simulink model "ML_UAV_3D_2"  (R2018a)
settings: Solver=ode4  StartTime=0.0  StopTime=130  FixedStep=Ts  MaxStep=2*T  MinStep=T  RelTol=1e-4
values from neighbouring files (symbols this model uses):
  Ac = 0.0331    [init_ML_UAV_3D_2.m]
  Am1_LPF = sysd.denominator{1}    [init_ML_UAV_3D_2.m]
  Am2_LPF = sysd.denominator{1}    [init_ML_UAV_3D_2.m]
  Am_coup_LPF = sysd.denominator{1}    [init_ML_UAV_3D_2.m]
  Amp_sf = 3    [init_ML_UAV_3D_2.m]
  Amp_sf_rp = 0.05*uav.m*g    [init_ML_UAV_3D_2.m]
  Bm1_LPF = sysd.numerator{1}    [init_ML_UAV_3D_2.m]
  Bm2_LPF = sysd.numerator{1}    [init_ML_UAV_3D_2.m]
  Bm_coup_LPF = sysd.numerator{1}    [init_ML_UAV_3D_2.m]
  C_S = [5;5;9]*10^-3    [init_ML_UAV_3D_2.m]
  Cd_u = 0.2    [init_ML_UAV_3D_2.m]
  dc_M_p = 6.7    [init_ML_UAV_3D_2.m]
  eps_V = 0.5    [init_ML_UAV_3D_2.m]
  g = 9.81    [init_ML_UAV_3D_2.m]
  gamma_d_p = (2*0.3/0.03*2*0.2*12/4)/10    (= 2.4)    [init_ML_UAV_3D_2.m]
  k3 = 24    [init_ML_UAV_3D_2.m]
  k4 = 0.8    [init_ML_UAV_3D_2.m]
  min_sf = 5    [init_ML_UAV_3D_2.m]
  min_sf_rp = 0.35*uav.m*g    [init_ML_UAV_3D_2.m]
  OMEGA_FILTER_OUTER = 40    [estimation.m]
  T_init = 10    [init_ML_UAV_3D_2.m]
  Tc = 1/500    (= 0.002)    [estimation.m]
  Tg = 1/ 20    (= 0.05)    [estimation.m]
  Tn = 1/500    (= 0.002)    [estimation.m]
  Ts = 1/500    (= 0.002)    [estimation.m]    (also in init_ML_UAV_3D_2.m)
  Tsc = 1/100    (= 0.01)    [estimation.m]
  Tz = 1/500    (= 0.002)    [estimation.m]
  X_GPS_offset = [0.01 0.005]    [estimation.m]
undefined symbols (not defined in the file or in its folder): Am_HPF, Am_LPF, Am_LPF2, an1, an1_v, an2, an3, Bm_HPF, Bm_LPF, Bm_LPF2, bn1, bn1_v, bn2, bn3, buoy, cable, controller, current, D_b, DiscIntNeverNeededParam, F, filters, J_u, K, kd_t, kp_t, L, Light, magnitude, MIL, Phi0, Psi0, R_b, T, Theta0, theta_q_ini, tolerences, torque_corr, uav, Vol_b, water, wave, X0_u
libraries: simulink x48, simulink_extras x10, UAV_Control x4, dspmtrx3 x2, aerolibwind2 x2
(part 6 of 6)

== system ML_UAV_3D_2/Quadrotor+buoy/6-DOF equations of motion Earth frame/azimuthal dynamics/Coupled System's azimuthal dynamics/elevation and azimuth angles dynamics in the coupled system ==
  alpha_phi_ddot : Inport
  alpha phi init : Inport  Port=2
  alpha_phi_dot init : Inport  Port=3
  reset : Inport  Port=4
  Enable : EnablePort
  " alpha" : Scope
  " alpha dot" : Scope
  " alpha dot init" : Scope
  " alpha init" : Scope
  "alpha, phi" : DiscreteIntegrator  IntegratorMethod=Integration: Backward Euler  ExternalReset=level  InitialConditionSource=external  InitialCondition=a_p_0  SampleTime=-1  ICPrevOutput=DiscIntNeverNeededParam  ICPrevScaledInput=DiscIntNeverNeededParam
  "dot(alpha, phi)" : DiscreteIntegrator  IntegratorMethod=Integration: Backward Euler  ExternalReset=level  InitialConditionSource=external  SampleTime=-1  ICPrevOutput=DiscIntNeverNeededParam  ICPrevScaledInput=DiscIntNeverNeededParam
  "reset " : Scope
  "alpha, phi " : Outport
  "alpha_dot, phi_dot" : Outport  Port=2
  wires:
  "dot(alpha, phi)"/1 -> "alpha, phi"/1, " alpha dot"/1, "alpha_dot, phi_dot"/1
  alpha_phi_ddot/1 -> "dot(alpha, phi)"/1
  "alpha, phi"/1 -> "alpha, phi "/1, " alpha"/1
  alpha_phi_dot init/1 -> " alpha dot init"/1, "dot(alpha, phi)"/3
  alpha phi init/1 -> " alpha init"/1, "alpha, phi"/3
  reset/1 -> "reset "/1, "alpha, phi"/2, "dot(alpha, phi)"/2

== system ML_UAV_3D_2/Quadrotor+buoy/6-DOF equations of motion Earth frame/azimuthal dynamics/Coupled System's azimuthal dynamics/get initial elevation and azimuth angle for the coupled dynamics ==
  "alpha, phi decoupled" : Inport
  "alpha_dot, phi_dot decoupled" : Inport  Port=2
  Trigger : TriggerPort  VariantControl=Variant
  "alpha, phi init" : Outport
  "alpha_dot, phi_dot init" : Outport  Port=2
  wires:
  "alpha, phi decoupled"/1 -> "alpha, phi init"/1
  "alpha_dot, phi_dot decoupled"/1 -> "alpha_dot, phi_dot init"/1

== system ML_UAV_3D_2/Quadrotor+buoy/6-DOF equations of motion Earth frame/azimuthal dynamics/Decoupled System's elevation and azimuth dynamics/elevation and azimuth angles to Direction Cosine Matrix Spherical to Cartesian ==
  "alpha, phi" : Inport
  -s_alpha*c_phi : Fcn  Expr=-u(1)*u(4)
  -s_alpha*s_phi : Fcn  Expr=-u(1)*u(2)
  -s_phi : Fcn  Expr=-u(2)
  Ground : Ground
  Mux : Mux  Inputs=2
  Subsystem : Subsystem
  c_alpha : Fcn  Expr=u(3)
  c_alpha*c_phi : Fcn  Expr=u(3)*u(4)
  c_alpha*s_phi : Fcn  Expr=u(3)*u(2)
  c_phi : Fcn  Expr=u(4)
  s_alpha : Fcn  Expr=u(1)
  sincos : Trigonometry  Operator=sincos
  DCM : Outport  PortDimensions=[3,3]
  wires:
  -s_alpha*c_phi/1 -> Subsystem/2(In2)
  -s_phi/1 -> Subsystem/3(In3)
  Subsystem/1(Out1) -> DCM/1
  c_alpha/1 -> Subsystem/8(In8)
  sincos/2 -> Mux/2
  s_alpha/1 -> Subsystem/7(In7)
  c_alpha*s_phi/1 -> Subsystem/4(In4)
  Ground/1 -> Subsystem/9(In9)
  Mux/1 -> c_alpha*s_phi/1, s_alpha/1, c_alpha/1, c_phi/1, -s_alpha*s_phi/1, -s_phi/1, -s_alpha*c_phi/1, c_alpha*c_phi/1
  -s_alpha*s_phi/1 -> Subsystem/5(In5)
  c_alpha*c_phi/1 -> Subsystem/1(In1)
  c_phi/1 -> Subsystem/6(In6)
  sincos/1 -> Mux/1
  "alpha, phi"/1 -> sincos/1

== system ML_UAV_3D_2/Quadrotor+buoy/6-DOF equations of motion Earth frame/azimuthal dynamics/Decoupled System's elevation and azimuth dynamics/magnitude ==
  dX : Inport
  Math Function2 : Math  Operator=square  SaturateOnIntegerOverflow=on
  Sqrt : Sqrt  SaturateOnIntegerOverflow=on
  Sum of Elements : Sum  Inputs=+
  r : Outport
  wires:
  Math Function2/1 -> Sum of Elements/1
  Sum of Elements/1 -> Sqrt/1
  dX/1 -> Math Function2/1
  Sqrt/1 -> r/1

== system ML_UAV_3D_2/Quadrotor+buoy/6-DOF equations of motion Earth frame/azimuthal dynamics/Decoupled System's elevation and azimuth dynamics/magnitude1 ==
  dX : Inport
  Math Function2 : Math  Operator=square  SaturateOnIntegerOverflow=on
  Sqrt : Sqrt  SaturateOnIntegerOverflow=on
  Sum of Elements : Sum  Inputs=+
  r : Outport
  wires:
  Sqrt/1 -> r/1
  dX/1 -> Math Function2/1
  Sum of Elements/1 -> Sqrt/1
  Math Function2/1 -> Sum of Elements/1

== system ML_UAV_3D_2/Sensors and Filters/Sensors/ Sonar (10Hz) (true elevation instead real sonar signal)/Sampler/Triggered Subsystem ==
  In1 : Inport
  Trigger : TriggerPort  VariantControl=(inherit)
  Out1 : Outport
  wires:
  In1/1 -> Out1/1

== system ML_UAV_3D_2/UAV controller/u_r_p_Lyapunov radial position2/output conditioning/Subsystem1/ur smooth lower bound, coupled ==
  u : Inport
  Manual Switch : ManualSwitch
  Mux3 : Mux  Inputs=2
  Saturation1 : Saturate  UpperLimit=inf  LowerLimit=min_sf
  apply for lower bound only : Switch  Criteria=u2 > Threshold  Threshold=Amp_sf+min_sf
  sat : Scope
  saturation function : Fcn  Expr=Amp_sf*tanh((u(1)-(Amp_sf+min_sf))/(Amp_sf)) + (Amp_sf+min_sf)
  sat(u) : Outport
  wires:
  Manual Switch/1 -> sat(u)/1
  Saturation1/1 -> Manual Switch/2
  u/1 -> saturation function/1, apply for lower bound only/2, Mux3/1, apply for lower bound only/1, Saturation1/1
  saturation function/1 -> apply for lower bound only/3, Mux3/2
  Mux3/1 -> sat/1
  apply for lower bound only/1 -> Manual Switch/1

== system ML_UAV_3D_2/UAV controller/u_r_p_Lyapunov radial position2/output conditioning/Subsystem1/ur smooth lower bound, decoupled ==
  u : Inport
  Manual Switch : ManualSwitch
  Mux3 : Mux  Inputs=2
  Saturation1 : Saturate  UpperLimit=inf  LowerLimit=min_sf_rp
  apply for lower bound only : Switch  Criteria=u2 > Threshold  Threshold=Amp_sf_rp+min_sf_rp
  sat : Scope
  saturation function : Fcn  Expr=Amp_sf_rp*tanh((u(1)-(Amp_sf_rp+min_sf_rp))/(Amp_sf_rp)) + (Amp_sf_rp+min_sf_rp)
  sat(u) : Outport
  wires:
  Manual Switch/1 -> sat(u)/1
  Saturation1/1 -> Manual Switch/2
  u/1 -> saturation function/1, apply for lower bound only/2, Mux3/1, apply for lower bound only/1, Saturation1/1
  saturation function/1 -> apply for lower bound only/3, Mux3/2
  Mux3/1 -> sat/1
  apply for lower bound only/1 -> Manual Switch/1

== system ML_UAV_3D_2/UAV controller/u_r_p_Lyapunov radial position2/output conditioning/smooth switching with memory/Enabled Subsystem1 ==
  In1 : Inport
  Enable : EnablePort
  Out1 : Outport
  wires:
  In1/1 -> Out1/1

== system ML_UAV_3D_2/UAV controller/u_r_p_Lyapunov radial position2/output conditioning/smooth switching with memory/Enabled Subsystem2 ==
  In1 : Inport
  Enable : EnablePort
  Out1 : Outport
  wires:
  In1/1 -> Out1/1

== system ML_UAV_3D_2/UAV controller/u_r_p_Lyapunov radial position2/output conditioning/smooth switching with memory/smooth switch ==
  note: if switch == 0
      | y = u2
      | elseif switch == 1
      | y = u1
      | end
  u 1 : Inport
  u 2 : Inport  Port=2
  switch : Inport  Port=3
  Constant : Constant
  Data Type Conversion : DataTypeConversion
  Low Pass Filter2 : DiscreteTransferFcn  Numerator=filters.Bm_coup_LPF  Denominator=filters.Am_coup_LPF
  Product : Product
  Product1 : Product
  Step1 : Step  SampleTime=0
  Subtract : Sum  Inputs=+-
  Sum : Sum  Inputs=|++
  "switch " : Scope
  y : Outport
  wires:
  Product/1 -> Sum/2
  Product1/1 -> Sum/1
  Low Pass Filter2/1 -> "switch "/1, Product/1, Subtract/2
  Data Type Conversion/1 -> Low Pass Filter2/1
  u 2/1 -> Product1/1
  u 1/1 -> Product/2
  switch/1 -> Data Type Conversion/1
  Sum/1 -> y/1
  Constant/1 -> Subtract/1
  Subtract/1 -> Product1/2

== system ML_UAV_3D_2/UAV controller/u_r_p_Lyapunov radial position3/output conditioning/Subsystem1/ur smooth lower bound, coupled ==
  u : Inport
  Manual Switch : ManualSwitch
  Mux3 : Mux  Inputs=2
  Saturation1 : Saturate  UpperLimit=inf  LowerLimit=min_sf
  apply for lower bound only : Switch  Criteria=u2 > Threshold  Threshold=Amp_sf+min_sf
  sat : Scope
  saturation function : Fcn  Expr=Amp_sf*tanh((u(1)-(Amp_sf+min_sf))/(Amp_sf)) + (Amp_sf+min_sf)
  sat(u) : Outport
  wires:
  Manual Switch/1 -> sat(u)/1
  Saturation1/1 -> Manual Switch/2
  u/1 -> saturation function/1, apply for lower bound only/2, Mux3/1, apply for lower bound only/1, Saturation1/1
  saturation function/1 -> apply for lower bound only/3, Mux3/2
  Mux3/1 -> sat/1
  apply for lower bound only/1 -> Manual Switch/1

== system ML_UAV_3D_2/UAV controller/u_r_p_Lyapunov radial position3/output conditioning/Subsystem1/ur smooth lower bound, decoupled ==
  u : Inport
  Manual Switch : ManualSwitch
  Mux3 : Mux  Inputs=2
  Saturation1 : Saturate  UpperLimit=inf  LowerLimit=min_sf_rp
  apply for lower bound only : Switch  Criteria=u2 > Threshold  Threshold=Amp_sf_rp+min_sf_rp
  sat : Scope
  saturation function : Fcn  Expr=Amp_sf_rp*tanh((u(1)-(Amp_sf_rp+min_sf_rp))/(Amp_sf_rp)) + (Amp_sf_rp+min_sf_rp)
  sat(u) : Outport
  wires:
  Manual Switch/1 -> sat(u)/1
  Saturation1/1 -> Manual Switch/2
  u/1 -> saturation function/1, apply for lower bound only/2, Mux3/1, apply for lower bound only/1, Saturation1/1
  saturation function/1 -> apply for lower bound only/3, Mux3/2
  Mux3/1 -> sat/1
  apply for lower bound only/1 -> Manual Switch/1

== system ML_UAV_3D_2/UAV controller/u_r_p_Lyapunov radial position3/output conditioning/smooth switching with memory/Enabled Subsystem1 ==
  In1 : Inport
  Enable : EnablePort
  Out1 : Outport
  wires:
  In1/1 -> Out1/1

== system ML_UAV_3D_2/UAV controller/u_r_p_Lyapunov radial position3/output conditioning/smooth switching with memory/Enabled Subsystem2 ==
  In1 : Inport
  Enable : EnablePort
  Out1 : Outport
  wires:
  In1/1 -> Out1/1

== system ML_UAV_3D_2/UAV controller/u_r_p_Lyapunov radial position3/output conditioning/smooth switching with memory/smooth switch ==
  note: if switch == 0
      | y = u2
      | elseif switch == 1
      | y = u1
      | end
  u 1 : Inport
  u 2 : Inport  Port=2
  switch : Inport  Port=3
  Constant : Constant
  Data Type Conversion : DataTypeConversion
  Low Pass Filter2 : DiscreteTransferFcn  Numerator=Bm_coup_LPF  Denominator=Am_coup_LPF
  Product : Product
  Product1 : Product
  Step1 : Step  SampleTime=0
  Subtract : Sum  Inputs=+-
  Sum : Sum  Inputs=|++
  "switch " : Scope
  y : Outport
  wires:
  Product/1 -> Sum/2
  Product1/1 -> Sum/1
  Low Pass Filter2/1 -> "switch "/1, Product/1, Subtract/2
  Data Type Conversion/1 -> Low Pass Filter2/1
  u 2/1 -> Product1/1
  u 1/1 -> Product/2
  switch/1 -> Data Type Conversion/1
  Sum/1 -> y/1
  Constant/1 -> Subtract/1
  Subtract/1 -> Product1/2

== system ML_UAV_3D_2/Quadrotor+buoy/6-DOF equations of motion Earth frame/azimuthal dynamics/Decoupled System's elevation and azimuth dynamics/elevation and azimuth angles to Direction Cosine Matrix Spherical to Cartesian/Subsystem ==
  In1 : Inport
  In2 : Inport  Port=2
  In3 : Inport  Port=3
  In4 : Inport  Port=4
  In5 : Inport  Port=5
  In6 : Inport  Port=6
  In7 : Inport  Port=7
  In8 : Inport  Port=8
  In9 : Inport  Port=9
  Matrix Concatenate : Concatenate  NumInputs=3  Mode=Multidimensional array  ConcatenateDimension=2
  Mux : Mux  Inputs=3
  Mux1 : Mux  Inputs=3
  Mux2 : Mux  Inputs=3
  Reshape : Reshape  OutputDimensionality=Column vector (2-D)
  Reshape1 : Reshape  OutputDimensionality=Column vector (2-D)
  Reshape2 : Reshape  OutputDimensionality=Column vector (2-D)
  Out1 : Outport
  wires:
  Reshape1/1 -> Matrix Concatenate/2
  Mux1/1 -> Reshape1/1
  Reshape/1 -> Matrix Concatenate/1
  Reshape2/1 -> Matrix Concatenate/3
  Matrix Concatenate/1 -> Out1/1
  Mux2/1 -> Reshape2/1
  In1/1 -> Mux/1
  Mux/1 -> Reshape/1
  In4/1 -> Mux/2
  In7/1 -> Mux/3
  In2/1 -> Mux1/1
  In8/1 -> Mux1/3
  In5/1 -> Mux1/2
  In3/1 -> Mux2/1
  In6/1 -> Mux2/2
  In9/1 -> Mux2/3

== matlab function ML_UAV_3D_2/Sea2/Water current ==
  data: Uc input; Us input; uc output; beta input; psi_b input; vc output; psi_w input
function [uc,vc] = fcn(Uc,Us,beta,psi_b,psi_w)

%% body frame:
% uc = Uc*cos(beta - psi_b) + sum( Us.*cos(psi_w - psi_b) );
% vc = Uc*sin(beta - psi_b) + sum( Us.*sin(psi_w - psi_b) );

%% inertial frame:
uc = Uc*cos(beta) + sum( Us.*cos(psi_w) );
vc = Uc*sin(beta) + sum( Us.*sin(psi_w) );

== matlab function ML_UAV_3D_2/Quadrotor+buoy/6-DOF equations of motion Earth frame/Coupling state/MATLAB Function ==
  data: pos_T input; is_coupled output; re_couple input; coupled input; c output
function [is_coupled,c] = fcn(pos_T, re_couple, coupled)

% persistent coupled
% if isempty(coupled) 
%     coupled = 1;
% end

if and(pos_T == 1 , coupled == 1)
    coupled = 1;
    c = 1; 
    
elseif and(pos_T == 0 , coupled == 1)
    coupled = 0;
    c = 2;
elseif and(coupled == 0 , re_couple == 0)
    coupled = 0;
    c = 3;
elseif and(coupled == 0 , re_couple == 1)
    coupled = 1;
    c = 4;
elseif and(pos_T == 0 , coupled == 0)
    coupled = 0;
    c = 5;
else
    coupled = 1;
    c = 6;
end
    
is_coupled = coupled;

== matlab function ML_UAV_3D_2/Sensors and Filters/Data processing/Estimate Attitude/Kalman Filter - Pitch ==
  settings: updateMethod=DISCRETE  sampleTime=T
  data: angle output; acc_angle input; gyro_rate input; opti_angle input; dt input
function angle   = fcn(acc_angle,gyro_rate,opti_angle,dt)
%#eml
    % a bias in the accelerometer will result in a bias in the filter
    % estimate
    Q_angle = 0.001;
    Q_gyro   = 0.001; %0.01;  %0.003
    R_angle  =  0.01;  %0.03

    
    persistent P_00;
    persistent P_01;
    persistent P_10;
    persistent P_11;
    persistent x_angle;
    persistent x_bias;
        
    if isempty(P_00)
        P_00 = 1.5*10^-4;
    end
    
    if isempty(P_01)
        P_01 = -1.4*10^-4;
    end
    if isempty(P_10)
        P_10 = -1.4*10^-4;
    end
    if isempty(P_11)
        P_11 = 11.4*10^-4;
    end
     if isempty(x_bias)
        x_bias = 0;
     end
     if isempty(x_angle)
        x_angle = 0;
     end
    
    
    % Calculate the new output
    x_angle = x_angle + dt * (gyro_rate - x_bias);%
    P_00 = P_00 -  dt * (P_10 + P_01) + Q_angle * dt;
    P_01 = P_01  - dt * P_11;
    P_10 = P_10  - dt * P_11;
    P_11 = P_11  + Q_gyro * dt;

    % Assuming H = [0.98 (effect of gyro) 0.02 (effect of acc)]
    %e = (0.97*x_angle + 0.03*acc_angle) - x_angle;
    e = (0.9*x_angle + 0.001*acc_angle + 0.099*opti_angle) - x_angle;
    S = P_00 + R_angle;
    K_0 = P_00 / S;
    K_1 = P_10 / S;

    % Correction
    x_angle = x_angle+  K_0 * e;
    x_bias  = x_bias+  K_1 * e;
    P_00 = P_00 - K_0 * P_00;
    P_01 = P_01 - K_0 * P_01;
    P_10 = P_10 - K_1 * P_00;
    P_11 = P_11 - K_1 * P_01;

    angle = x_angle;
%     P = [P_00 P_01; P_10 P_11];

== matlab function ML_UAV_3D_2/Sensors and Filters/Coupling detection by r/Coupling state/MATLAB Function ==
  data: pos_T input; is_coupled output; re_couple input; coupled input; c output
function [is_coupled,c] = fcn(pos_T, re_couple, coupled)

% persistent coupled
% if isempty(coupled) 
%     coupled = 1;
% end

if and(pos_T == 1 , coupled == 1)
    coupled = 1;
    c = 1; 
    
elseif and(pos_T == 0 , coupled == 1)
    coupled = 0;
    c = 2;
elseif and(coupled == 0 , re_couple == 0)
    coupled = 0;
    c = 3;
elseif and(coupled == 0 , re_couple == 1)
    coupled = 1;
    c = 4;
elseif and(pos_T == 0 , coupled == 0)
    coupled = 0;
    c = 5;
else
    coupled = 1;
    c = 6;
end
    
is_coupled = coupled;

== matlab function ML_UAV_3D_2/Sensors and Filters/Data processing/Estimate Position/Extrapolation - x ==
  settings: updateMethod=DISCRETE
  data: xin input; xout output; xdotin input; dt input; new input; isTracking input; x0 input
function xout = fcn(xin, xdotin, dt, new, isTracking,x0)
%#codegen

%
% Pass through input if "new" data available and OptiTrack is tracking.
% Otherwise, use linear interpolation to estimate the signal value and
% ignore the input data.
%
persistent x;

if( isempty(x) )
    x = x0;
end;

if( new == 1 && isTracking == 1 )
    x = xin;
else
    x = x+dt*xdotin;
end;

xout = x;

== matlab function ML_UAV_3D_2/Preprocessing Unit/setpoint velocity controller  ==
  settings: updateMethod=DISCRETE
  data: V_ref input; phi_bar input; Vb input; r_ref input; alpha_ref output; zb input; phi_bar_dec output; zu_ref input; D_b11 input; T_bar output
function [alpha_ref,phi_bar_dec,T_bar] = ...
    fcn(V_ref, phi_bar,Vb,r_ref,zb,zu_ref,D_b11)

% if t < 1
%     r_ref = 3; %r_0 = 3;
% else
%     r_ref = 6.7; %r_bar = 6.7;
% end

alpha_ref = asin( (zu_ref - zb)/r_ref );

xb_dot_ref = V_ref*cos(phi_bar);
yb_dot_ref = V_ref*sin(phi_bar);

% phi_bar_dec = atan2( V_ref*sin(psi_V_ref)-Vb(2), V_ref*cos(psi_V_ref)-Vb(1));
phi_bar_dec = phi_bar;

% mag2_Vb = sqrt(Vb(1)^2 + Vb(2)^2);
T_bar = D_b11*sqrt( (xb_dot_ref-Vb(1))^2 + (yb_dot_ref-Vb(2))^2 )/cos(alpha_ref);

== matlab function ML_UAV_3D_2/Sensors and Filters/Data processing/Estimate Position/Extrapolation - z ==
  settings: updateMethod=DISCRETE  sampleTime=T
  data: xin input; xout output; xdotin input; dt input; new input; isTracking input; x0 input
function xout = fcn(xin, xdotin, dt, new, isTracking,x0)
%#codegen

%
% Pass through input if "new" data available and OptiTrack is tracking.
% Otherwise, use linear interpolation to estimate the signal value and
% ignore the input data.
%
persistent x;

if( isempty(x) )
    x = x0;
end

if( new == 1 && isTracking == 1 )
    x = xin;
else
    x = x+dt*xdotin;
end

xout = x;

== matlab function ML_UAV_3D_2/UAV controller/cond1/MATLAB Function ==
  settings: updateMethod=DISCRETE
  data: r input; r_dot input; y output; coupled input; Lc input; dt input; t output
function [y,t]  = fcn(r,r_dot,coupled,Lc,dt)

persistent key
persistent timer

if isempty(key)
    key = 0;
end

if isempty(timer)
    timer = 0;
end

if (r > Lc - 0.1) && (r_dot > 0.25) && (key == 0)
    key = 1;
end

if (r < Lc - 0.12) && (r_dot < -0.1) && (key == 1)
    key = 0;
end

if (key == 1) && (coupled == 1)
    timer = timer + dt;
end

if (timer >= 1) % reset
    key = 0;
    timer = 0;
end

y = key;
t = timer;

== matlab function ML_UAV_3D_2/Preprocessing Unit/Damping Coefficient Calculation ==
  settings: updateMethod=DISCRETE
  data: Re output; V_bar input; delta_h input; h_b input; l_b input; C_S_bar output; rho input; nu input; b_11 input; D11_0 output
function [Re,C_S_bar,D11_0]  = fcn(V_bar,delta_h,h_b,l_b,rho,nu,b_11)

Re = max(abs(V_bar)*l_b/nu,0.5*10^5);

C_S_bar = 0.075/(log10(Re) -2 )^2;

D11_0 = V_bar*( max(min(delta_h+h_b/2,h_b),0)*(2*l_b) + (l_b*h_b) )...
        *0.5*rho*C_S_bar + b_11;

== matlab function ML_UAV_3D_2/UAV controller/State Machine new ==
  settings: updateMethod=DISCRETE  sampleTime=T
  data: eps input; r input; r_thr input; active output; mag_Vb2 input; psi_Vb input; V_bar0 input; c output; V_bar input; reset input
function [active,c] = fcn(eps,r, r_thr,mag_Vb2,psi_Vb, V_bar0, V_bar,reset)

persistent state
persistent is_active

if isempty(is_active) 
    state = 0;
    is_active = 0;
end

eps = abs(eps); % make sure that eps is positive.
eps_p1 = 2*eps;
eps_p2 = 2.5*eps;
eps_n1 = 1.5*eps;
eps_n2 = 2*eps;

dx_thr = 0.13;  
% deactivate the velocity controller while reset is on:
if (reset == 1)
    is_active = 0;
    % idel state
    state = 0; 
% buoy velocity is low, activate to accelerate:
elseif and( is_active == 0, mag_Vb2 <= V_bar0-eps_n1 )  
    is_active = 1;
    % accelerate flag state
    state = 1;     
 
% deactivate since velocity has gone too high or the system has
% unintentionnally decouple to prevent damage (removed for testing):
elseif and( is_active == 1 , (mag_Vb2 >= V_bar+eps_p1) ) % (r < r_thr)
    is_active = 0;
    % acceleration stop state
    state = 2;
    
% deactivate since velocity has gone too high or the system has
% unintentionnally decouple to prevent damage:
% elseif and( is_active == 1, or( (mag_Vb2 >= V_bar+eps_n1), (r < r_thr) )) % (r < r_thr)
%     is_active = 0;
%     % acceleration stop state
%     state = 3; 
end    
 
%%
c           = state;
active      =  is_active;

== matlab function ML_UAV_3D_2/Refenrence Commands/setpoint velocity controller1 ==
  settings: updateMethod=DISCRETE
  data: eps input; r input; er_thr input; V_bar_out output; phi_bar_out output; Lc0 input; c output; V0_bar input; phi0_bar input; V input
function [V_bar_out,phi_bar_out,c] = fcn(eps,r, er_thr, Lc0,...
            V0_bar,phi0_bar, V) 

persistent V0_old
if isempty(V0_old) 
    V0_old = 0;
end

eps = abs(eps); % make sure that eps is positive.

% Velocity error is low, no output.
if (V0_bar - V <  eps) && (V0_bar - V >=  0)
    V_bar_out = V0_old;
    % return previous V0
    c = 0; 
% Velocity error is high, output the velocity only if the UAV is ready.
elseif (V0_bar - V >=  eps) && (Lc0 - r < er_thr)
    V_bar_out = V0_bar;
    % follow new V0
    c = 1;     
% Velocity error is low, no output.
elseif (V0_bar - V >  -eps) && (V0_bar - V <  0)
    V_bar_out = V0_old;
    % return previous V0
    c = 2; 
% Velocity error is high, output the velocity only if the UAV is ready.
elseif (V0_bar - V <=  -eps) && (Lc0 - r < er_thr)
    V_bar_out = V0_bar;
    % follow new V0
    c = 3;
else  % Velocity error is high, but UAV is not ready
    V_bar_out = V0_old;
    c = 4;
end

% when the new reference velocity is sent to the ouptut,
% set the old reference velocity to the current reference velocty
% to be the zero point when the reference velocty changes again.
if  V_bar_out == V0_bar
    V0_old = V0_bar;
end

phi_bar_out = phi0_bar;

== matlab function ML_UAV_3D_2/UAV controller/Attitutde Control/PID control law with saturation and ff acceleration1 ==
  settings: updateMethod=DISCRETE
  data: ex input; ex_int output; u output; ex_dot input; xd_ddot input; kp input; kd input; ki input; exi_max input; u_min input; u_max input; m input; dt input; u_sat output
function [ex_int,u,u_sat] = fcn(ex,ex_dot,xd_ddot,kp,kd,ki,exi_max,u_min,u_max,m,dt)

persistent int_ex;

if isempty(int_ex)
    int_ex = 0;
end

int_ex = max(min(int_ex + ex*dt,exi_max),-exi_max);

u = m*(-kp*ex - ki*int_ex - kd*ex_dot + xd_ddot);

u_sat = max(min(u,u_max),u_min);

ex_int = int_ex;

== matlab function ML_UAV_3D_2/UAV controller/Attitutde Control/PID control law with saturation and ff acceleration ==
  settings: updateMethod=DISCRETE
  data: ex input; ex_int output; u output; ex_dot input; xd_ddot input; kp input; kd input; ki input; exi_max input; u_min input; u_max input; m input; dt input; u_sat output
function [ex_int,u,u_sat] = fcn(ex,ex_dot,xd_ddot,kp,kd,ki,exi_max,u_min,u_max,m,dt)

persistent int_ex;

if isempty(int_ex)
    int_ex = 0;
end

int_ex = max(min(int_ex + ex*dt,exi_max),-exi_max);

u = m*(-kp*ex - ki*int_ex - kd*ex_dot + xd_ddot);

u_sat = max(min(u,u_max),u_min);

ex_int = int_ex;

== matlab function ML_UAV_3D_2/UAV controller/Decoupling control signals /control signals decoupling ==
  data: ur input; u_C output; u1 output; phi_u output; theta_u output; ua input; uf input; alpha input; phi input; psi_u input; uz_min input; u1_max input; tilt_max input
function [u_C,u1,phi_u,theta_u] = fcn(ur,ua,uf,alpha,phi,psi_u,...
            uz_min,u1_max,tilt_max)

% u_C = [ux;uy;uz]
% tested for correctness

u_C = [cos(alpha)*cos(phi),  -sin(alpha)*cos(phi), -sin(phi)
       cos(alpha)*sin(phi),  -sin(alpha)*sin(phi),  cos(phi)
       sin(alpha)         ,   cos(alpha)         ,     0    ]...
      ...
      *[ur;ua;uf];

u_C(3,1) = max(uz_min,u_C(3,1)); 

     u1 = min(sqrt(u_C(1,1)^2 + u_C(2,1)^2 + u_C(3,1)^2), u1_max);
     
  phi_u = atan( (u_C(1,1)*sin(psi_u) - u_C(2,1)*cos(psi_u)) / u_C(3,1) );
  
theta_u = asin( (u_C(1,1)*cos(psi_u) + u_C(2,1)*sin(psi_u)) /u1 );

  phi_u  = tilt_max*tanh(   phi_u/tilt_max );
theta_u  = tilt_max*tanh( theta_u/tilt_max );

== matlab function ML_UAV_3D_2/UAV controller/Attitutde Control/PID control law with saturation and ff acceleration2 ==
  settings: updateMethod=DISCRETE  sampleTime=Ts
  data: ex input; ex_int output; u output; ex_dot input; xd_ddot input; kp input; kd input; ki input; exi_max input; u_min input; u_max input; m input; dt input; u_sat output
function [ex_int,u,u_sat] = fcn(ex,ex_dot,xd_ddot,kp,kd,ki,exi_max,u_min,u_max,m,dt)

persistent int_ex;

if isempty(int_ex)
    int_ex = 0;
end

int_ex = max(min(int_ex + ex*dt,exi_max),-exi_max);

u = m*(-kp*ex - ki*int_ex - kd*ex_dot + xd_ddot);

u_sat = max(min(u,u_max),u_min);

ex_int = int_ex;

== matlab function ML_UAV_3D_2/Sensors and Filters/Data processing/Estimate Attitude/Calculate Roll and Pitch (From Acceleration Data)/calc_roll_pitch ==
  data: roll_acc output; pitch_acc output; acc_body input
function [roll_acc, pitch_acc]   = fcn(acc_body)
%#eml
n = norm(acc_body,2);
if n>eps
    acc_body = -acc_body/n; 
else
    acc_body = [0 0 1]';
end

roll_acc = atan2(acc_body(2),acc_body(3));
pitch_acc = atan2( -acc_body(1), acc_body(2)*sin(roll_acc)+acc_body(3)*cos(roll_acc));

== matlab function ML_UAV_3D_2/Sensors and Filters/Data processing/Estimate Position/Kalman Filter - Height ==
  settings: updateMethod=DISCRETE  sampleTime=T
  data: height output; optitrack input; sonar_d input; dt input; x0 input
function height   = fcn(optitrack,sonar_d,dt,x0)
%#eml

     Q_sonar  = 0.1; %0.01; %0.001
     Q_optitrack   = 0.01; %0.01;  %0.003
     R_height =  0.03;  %0.03

    
    persistent P_00;
    persistent P_01;
    persistent P_10;
    persistent P_11;
    persistent x_height;
    persistent x_bias;
        
    if isempty(P_00)
        P_00 = 0;
    end
    
    if isempty(P_01)
        P_01 = 0;
    end
    if isempty(P_10)
        P_10 = 0;
    end
    if isempty(P_11)
        P_11 = 0;
    end
    if isempty(x_bias)
       x_bias = 0;
    end
    if isempty(x_height)
       x_height = x0;
    end
    
    
    % Compensate for sonar rate calculation (sonar sample rate is 10Hz)
    sonar_d_corrected = sonar_d*dt*10;  % m/s
    
    % Reject large height rate changes from sonar
    % As those are likely a result of obstacle underneath or noise
    if(abs(sonar_d_corrected) > 1 )    % max height rate (m/s)
        sonar_d_corrected = 0;
    end
    
    % Calculate the new output
    %x_height = x_height + dt * (sonar_d - x_bias); % old 
    x_height = x_height + dt * (sonar_d_corrected - x_bias);
    P_00 = P_00 -  dt * (P_10 + P_01) + Q_sonar * dt;
    P_01 = P_01  - dt * P_11;
    P_10 = P_10  - dt * P_11;
    P_11 = P_11  + Q_optitrack * dt;

    % Assuming H = [0.95 (effect of optitrack) 0.05 (effect of sonar)]
    e = (0.05*x_height + 0.95*optitrack) - x_height;
    S = P_00 + R_height;
    K_0 = P_00 / S;
    K_1 = P_10 / S;

    % Correction
    x_height = x_height+  K_0 * e;
    x_bias  = x_bias+  K_1 * e;
    P_00 = P_00 - K_0 * P_00;
    P_01 = P_01 - K_0 * P_01;
    P_10 = P_10 - K_1 * P_00;
    P_11 = P_11 - K_1 * P_01;

    height = x_height;

== matlab function ML_UAV_3D_2/Sea2/Waves (elevation and speed) ==
  data: x input; zeta_xy output; y input; z input; t input; A input; psi input; omega input; k input; epsilon input; uw output; vw output; ww output; phi_water output; theta_water output
function [zeta_xy,uw,vw,ww,phi_water,theta_water] = ...
            fcn(x,y,z,t,A,psi,omega,k,epsilon)

f = - k*x.*cos(psi) - k.*y.*sin(psi) + omega*t + epsilon;
zeta_xy = sum( A.*sin(f) );

e = exp(k*z);

uw = sum( omega.*A.*e.*sin(f).*cos(psi) );
vw = sum( omega.*A.*e.*sin(f).*sin(psi) );
ww = sum( omega.*A.*e.*cos(f) );

  phi_water = atan( sum(-A.*k.*sin(psi).*cos(f)) );

theta_water = atan( sum(-A.*k.*cos(psi).*cos(f)) );

== matlab function ML_UAV_3D_2/Refenrence Commands/referense signals selector ==
  settings: updateMethod=DISCRETE
  data: V_ref input; phi_ref input; tv_ref input; V_ref_out output; r_ref input; phi_ref_out output; zu_ref input; tr_ref input; t input; r_ref_out output; zu_ref_out output
function [V_ref_out,phi_ref_out,r_ref_out,zu_ref_out] = ...
    fcn(V_ref,phi_ref,tv_ref,r_ref,zu_ref,tr_ref,t)

persistent i j

if isempty(i)
i = 1;
j = 1;
end

if i < length(V_ref-1)
    if t > tv_ref(i+1)
        i = i + 1;
    end
end

V_ref_out = V_ref(i);
phi_ref_out = phi_ref(i);

if j < length(r_ref-1)
    if t > tr_ref(j+1)
        j = j + 1;
    end
end

r_ref_out = r_ref(j);
zu_ref_out = zu_ref(j);

== matlab function ML_UAV_3D_2/UAV controller/MATLAB Function ==
  settings: updateMethod=DISCRETE  sampleTime=Ts
  data: eps input; active output; r input; r_thr input; mag_Vb2 input; psi_Vb input; V_bar0 input; V_bar input; reset input; c output
function [active,c] = fcn(eps,r, r_thr,mag_Vb2,psi_Vb, V_bar0, V_bar,reset)

persistent state
persistent is_active

if isempty(is_active) 
    state = 0;
    is_active = 0;
end

eps = abs(eps); % make sure that eps is positive.
eps_p1 = 2*eps;
eps_p2 = 2.5*eps;
eps_n1 = 1.5*eps;
eps_n2 = 2*eps;

dx_thr = 0.13;  
% deactivate the velocity controller while reset is on:
if (reset == 1)
    is_active = 0;
    % idel state
    state = 0; 
% buoy velocity is low, activate to accelerate:
elseif and( is_active == 0, mag_Vb2 <= V_bar0-eps_n1 )  
    is_active = 1;
    % accelerate flag state
    state = 1;     
 
% deactivate since velocity has gone too high or the system has
% unintentionnally decouple to prevent damage (removed for testing):
elseif and( is_active == 1 , (mag_Vb2 >= V_bar+eps_p1) ) % (r < r_thr)
    is_active = 0;
    % acceleration stop state
    state = 2;
    
% deactivate since velocity has gone too high or the system has
% unintentionnally decouple to prevent damage:
% elseif and( is_active == 1, or( (mag_Vb2 >= V_bar+eps_n1), (r < r_thr) )) % (r < r_thr)
%     is_active = 0;
%     % acceleration stop state
%     state = 3; 
end    
 
%%
c           = state;
active      =  is_active;

== matlab function ML_UAV_3D_2/Sensors and Filters/quadrotor position from relative buoy-UAV position/Buoy's States from UAV ==
  data: ru input; rb output; ru_dot input; ru_ddot input; R_S2C input; br input; br_dot input; br_ddot input; rb_dot output; rb_ddot output
function [rb,rb_dot,rb_ddot] = fcn(ru,ru_dot,ru_ddot,R_S2C,br,br_dot,br_ddot)

rb = ru - R_S2C*br;
rb_dot = ru_dot - R_S2C*br_dot;
rb_ddot = ru_ddot - R_S2C*br_ddot;

== matlab function ML_UAV_3D_2/Sensors and Filters/quadrotor position from relative buoy-UAV position/UAV's Spherical States ==
  data: r input; r_dot input; r_ddot input; alpha input; br output; alpha_dot input; alpha_ddot input; phi input; phi_dot input; br_dot output; br_ddot output; phi_ddot input; R_S2C output
function [br,br_dot,br_ddot,R_S2C] = fcn(r,r_dot,r_ddot,alpha,alpha_dot,...
        alpha_ddot,phi,phi_dot,phi_ddot)

br = [r;0;0];
    
br_dot = [r_dot; r*alpha_dot; r*cos(alpha)*phi_dot];


br_ddot = [r_ddot - r*alpha_dot^2 - r*(cos(alpha)*phi_dot)^2;
          r*alpha_ddot + 2*r_dot*alpha_dot + r*sin(alpha)*cos(alpha)*phi_dot^2;
          r*phi_ddot*cos(alpha)+2*r_dot*phi_dot*cos(alpha) - 2*r*alpha_dot*phi_dot*sin(alpha)];

R_S2C = [cos(alpha)*cos(phi) -sin(alpha)*cos(phi) -sin(phi)
         cos(alpha)*sin(phi) -sin(alpha)*sin(phi)  cos(phi)
         sin(alpha)           cos(alpha)             0     ];

== matlab function ML_UAV_3D_2/UAV controller/u_r_p_Lyapunov radial position2/MATLAB Function ==
  data: m_u input; r input; H output; PHI output; r_dot input; alpha input; alpha_dot input; phi input; phi_dot input; Xb_ddot input; psi_b input; nu_yb_dot input; cp input; pulling_flag input; b_inv output; Hc1 output; Hc2 output; Hc3 output; M_p output
function [H,PHI,b_inv,Hc1,Hc2,Hc3,M_p]   = fcn(m_u,r,r_dot,alpha,alpha_dot,phi,phi_dot,...
    Xb_ddot,psi_b,nu_yb_dot,cp, pulling_flag)


g = 9.81;

if pulling_flag == 0 % decoupled case:
    
    M_p = diag([1,r^2,r^2*cos(alpha)])*m_u;
    
    H_p = [ r*(alpha_dot^2 + cos(alpha)^2*phi_dot^2 ) ...
        - cos(alpha)*cos(phi)*Xb_ddot(1) - cos(alpha)*sin(phi)*Xb_ddot(2) ...
        - sin(alpha)*Xb_ddot(3) - g*sin(alpha);
        %
        r*(-2*r_dot*alpha_dot - r*sin(alpha)*cos(alpha)*phi_dot^2 ...
        + sin(alpha)*cos(phi)*Xb_ddot(1) + sin(alpha)*sin(phi)*Xb_ddot(2)...
        - cos(alpha)*Xb_ddot(3) - g*cos(alpha) );
        %
        r*( -2*r_dot*phi_dot*cos(alpha) + 2*r*alpha_dot*phi_dot*sin(alpha)...
        +sin(phi)*Xb_ddot(1) - cos(phi)*Xb_ddot(2) )
        ]*m_u;
    
    b_p_inv = diag([1,1/r,1/r]);
    
    %b_inv = diag([1,r,r*cos(alpha)])*m_u;
        
    PHI_p = [-1; 0; 0];
    
    M_p_inv = inv(M_p);
    
    H     = M_p_inv*H_p;  
    PHI   = M_p_inv*PHI_p; 
    b_inv = M_p*b_p_inv;
    
        Hc1 = 0;
        Hc2 = 0;
        Hc3 = 0;
else % coupled case:
    
    M_p = [   cos(alpha)*(cos(phi)*cos(psi_b) + sin(phi)*sin(psi_b)) 0 0
           -r*sin(alpha)*(cos(phi)*cos(psi_b) + sin(phi)*sin(psi_b))*0 r^2 0
                      -r*(sin(phi)*cos(psi_b) - cos(phi)*sin(psi_b))*0 0 r^2*cos(alpha) ]*m_u;
                  
    Hc1 = ( r*( alpha_dot^2 + cos(alpha)^2*phi_dot^2 ) ...
        + cos(alpha)*(cos(phi)*sin(psi_b) - sin(phi)*cos(psi_b))*nu_yb_dot...
        - sin(alpha)*Xb_ddot(3) )*cp - g*sin(alpha);
    
    Hc2 =   ( - r*sin(alpha)*cos(alpha)*phi_dot^2 ...
        - sin(alpha)*(cos(phi)*cos(psi_b) - sin(phi)*cos(psi_b))*nu_yb_dot...
        - cos(alpha)*Xb_ddot(3)  - g*cos(alpha) ); %*cp
    
    Hc3 = r*( 2*r*alpha_dot*phi_dot*sin(alpha) ...
          - (sin(phi)*sin(psi_b) + cos(phi)*cos(psi_b))*nu_yb_dot );
    
    
    H_p = [ Hc1; Hc2; Hc3]*m_u;
      

    % b_p = diag([1,r,r]) ;
    b_p_inv = diag([1,1/r,1/r]);
       
    PHI_p = [-1; 0; 0];
    
    M_p_inv = inv(M_p);
    
    H     = M_p_inv*H_p;  
    PHI   = M_p_inv*PHI_p; 
    b_inv = M_p*b_p_inv;

end


% syms r alpha phi
% 
% b = [cos(phi)/cos(alpha) 0  -sin(phi)
%      sin(phi)/cos(alpha) 0   cos(phi)
%      tan(alpha)/r        1/r 0       ];
% 
%  simplify(inv(b))
%     b_inv = [    cos(alpha)*cos(phi)    cos(alpha)*sin(phi)  0
%                 -sin(alpha)*cos(phi)   -sin(alpha)*sin(phi)  r
%                 -sin(phi)              cos(phi)             0  ];
%   simplify(inv(b_inv))

== matlab function ML_UAV_3D_2/UAV controller/u_r_p_Lyapunov radial position3/MATLAB Function ==
  data: m_u input; r input; H output; PHI output; r_dot input; alpha input; alpha_dot input; phi input; phi_dot input; phi_ddot input; Xb_ddot input; cp input; pulling_flag input; b_inv output
function [H,PHI,b_inv]   = fcn(m_u,r,r_dot,alpha,alpha_dot,phi,phi_dot,phi_ddot,...
    Xb_ddot,cp, pulling_flag)


g = 9.81;

if pulling_flag == 0 % decoupled case:
    
    H = [ r*(alpha_dot^2 + cos(alpha)^2*phi_dot^2 ) ...
        - cos(alpha)*cos(phi)*Xb_ddot(1) - cos(alpha)*sin(phi)*Xb_ddot(2) ...
        - sin(alpha)*Xb_ddot(3) - g*sin(alpha);
        %
        (-2*r_dot*alpha_dot - r*sin(alpha)*cos(alpha)*phi_dot^2 ...
        + sin(alpha)*cos(phi)*Xb_ddot(1) + sin(alpha)*sin(phi)*Xb_ddot(2)...
        - cos(alpha)*Xb_ddot(3) - g*cos(alpha) ) / r;
        %
        ( -2*r_dot*phi_dot*cos(alpha) + 2*r*alpha_dot*phi_dot*sin(alpha)...
        +sin(phi)*Xb_ddot(1) - cos(phi)*Xb_ddot(2) ) / (r*cos(alpha))
        ];
    
    b_inv = diag([1,r,r*cos(alpha)])*m_u;

    PHI = -[1/m_u
            0
            0];
        
else % coupled case:
    Hc1 = ( r*( alpha_dot^2 + cos(alpha)^2*phi_dot^2 ) ...
        - sin(alpha)*Xb_ddot(3) )*cp - g*sin(alpha);
    
    Hc2 =   ( - r*sin(alpha)*cos(alpha)*phi_dot^2 ...
        - cos(alpha)*Xb_ddot(3) )*cp - g*cos(alpha);
    
    Hc3 = ( -2*r*cos(alpha)*phi_ddot + 2*r*alpha_dot*phi_dot*sin(alpha) )*cp;
    
    
    H = [ cos(phi)/cos(alpha)*Hc1 - sin(phi)*Hc3;
          sin(phi)/cos(alpha)*Hc1 + cos(phi)*Hc3;
          tan(alpha)/r*Hc1 +          Hc2/r];
      
    b_inv = [    cos(alpha)*cos(phi)    cos(alpha)*sin(phi)  0
          -r*sin(alpha)*cos(phi) -r*sin(alpha)*sin(phi)  r^2
          r*sin(phi)             r*cos(phi)             0  ]*m_u;
      
    
    PHI = -[cos(phi)/cos(alpha)
            sin(phi)/cos(alpha)
            tan(alpha)/r       ]/m_u;
end


% syms r alpha phi
%
% b = [cos(phi)/cos(alpha) 0 -sin(phi)/r
%      sin(phi)/cos(alpha) 0  cos(phi)/r
%      tan(alpha)/r        1/r^2 0       ];
%
%  simplify(inv(b))

== matlab function ML_UAV_3D_2/UAV controller/u_r_p_Lyapunov radial position2/MATLAB Function2 ==
  data: phi input; e_phi output; phi_cmd input
function e_phi = fcn(phi, phi_cmd)

    e_phi = rem(phi - phi_cmd,2*pi);
    if e_phi > pi
        e_phi = e_phi - 2*pi;
    end
        if e_phi < -pi
        e_phi = e_phi + 2*pi;
        end
    
% if phi > 0 && phi_cmd > 0
%     e_phi = phi - phi_cmd;
%     
% elseif phi < 0 && phi_cmd < 0
%     e_phi = phi - phi_cmd;
%     
% elseif phi > 0 && phi_cmd < 0
%     e_phi = phi - phi_cmd
%     if e_phi > pi
%         e_phi = e_phi - 2*pi;
%     end
% elseif phi > 0 && phi_cmd < 0
%     if e_phi < pi
%         e_phi = e_phi + 2*pi;
%     end
% end

== matlab function ML_UAV_3D_2/UAV controller/u_r_p_Lyapunov radial position2/MATLAB Function4 ==
  data: Xb_ddot input; nu_b_dot output; psi_b input
function nu_b_dot = fcn(Xb_ddot,psi_b)

R_psi_b_inv = [ cos(psi_b) sin(psi_b)
               -sin(psi_b) cos(psi_b)];


nu_b_dot = R_psi_b_inv*[Xb_ddot(1); Xb_ddot(2)];

== matlab function ML_UAV_3D_2/Refenrence Commands/vector magnitude and angle1 ==
  settings: updateMethod=DISCRETE
  data: U2 input; mag_u2 output; direction2 output; psi_b input; nu_xb output; nu_yb output
function [mag_u2,direction2,nu_xb,nu_yb] = fcn(U2, psi_b) 

% U2 is a 2 elements' vector

mag_u2 = sqrt(sum(U2.^2));



direction2 = atan2( U2(2)+ eps, U2(1) + eps);

R_psi_b_inv = [ cos(psi_b) sin(psi_b)
               -sin(psi_b) cos(psi_b)];
           
nu_b = R_psi_b_inv*U2;

nu_xb = nu_b(1);
nu_yb = nu_b(2);
